simulink model "program_counter"  (R2020a)
settings: Solver=VariableStepAuto  StartTime=0.0  StopTime=10.0  RelTol=1e-3
libraries: simulink_extras x5
settings Model: Creator=F1  LastModifiedBy=F1

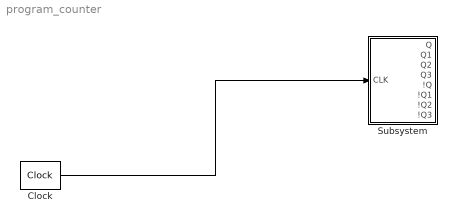
== system program_counter ==
  Clock : simulink_extras/Flip Flops/Clock  period=2
  Subsystem : Subsystem
  wires:
  Clock/1 -> Subsystem/1(CLK)

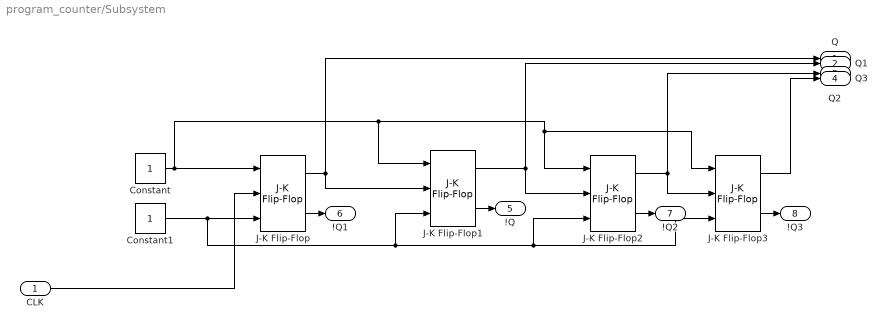
== system program_counter/Subsystem ==
  CLK : Inport
  Constant : Constant
  Constant1 : Constant
  J-K Flip-Flop{,1..3} (4 alike) : simulink_extras/Flip Flops/J-K Flip-Flop  initial_condition=0
  Q : Outport
  Q1 : Outport  Port=2
  Q2 : Outport  Port=3
  Q3 : Outport  Port=4
  !Q : Outport  Port=5
  !Q1 : Outport  Port=6
  !Q2 : Outport  Port=7
  !Q3 : Outport  Port=8
  wires:
  Constant1/1 -> J-K Flip-Flop3/3, J-K Flip-Flop2/3, J-K Flip-Flop1/3, J-K Flip-Flop/3
  J-K Flip-Flop1/1 -> Q1/1, J-K Flip-Flop2/2
  J-K Flip-Flop2/1 -> Q2/1, J-K Flip-Flop3/2
  Constant/1 -> J-K Flip-Flop/1, J-K Flip-Flop1/1, J-K Flip-Flop3/1, J-K Flip-Flop2/1
  J-K Flip-Flop/1 -> Q/1, J-K Flip-Flop1/2
  J-K Flip-Flop/2 -> !Q1/1
  J-K Flip-Flop1/2 -> !Q/1
  CLK/1 -> J-K Flip-Flop/2
  J-K Flip-Flop2/2 -> !Q2/1
  J-K Flip-Flop3/2 -> !Q3/1
  J-K Flip-Flop3/1 -> Q3/1
